simulink model "pv_panel_buck_converter_graphic"  (R2021a)
settings: Solver=VariableStepAuto  StartTime=0.0  StopTime=22  RelTol=1e-3  AbsTol=1e-3
libraries: spsSeriesRLCBranchLib x4, spsCurrentMeasurementLib x3, simulink x3, spsDiodeLib x1, spsMosfetLib x1, spsPVArrayLib x1, spsVoltageMeasurementLib x1, spspowerguiLib x1
settings Model: Creator=Uranus  LastModifiedBy=Uranus
settings SolverCC: AutoScaleAbsTol=off  AlgebraicLoopSolver=TrustRegion
settings DebuggingCC: SymbolicDimsDataTypeCodeGenerationDiagnostic=none  SFMachineParentedDataDiag=warning
settings SFSimCC: CustomCodeUndefinedFunction=UseInterfaceOnly
settings SimscapeCC: SimscapeLogType=all  SimscapeLogSimulationStatistics=on  SimscapeLogDataHistory=10000

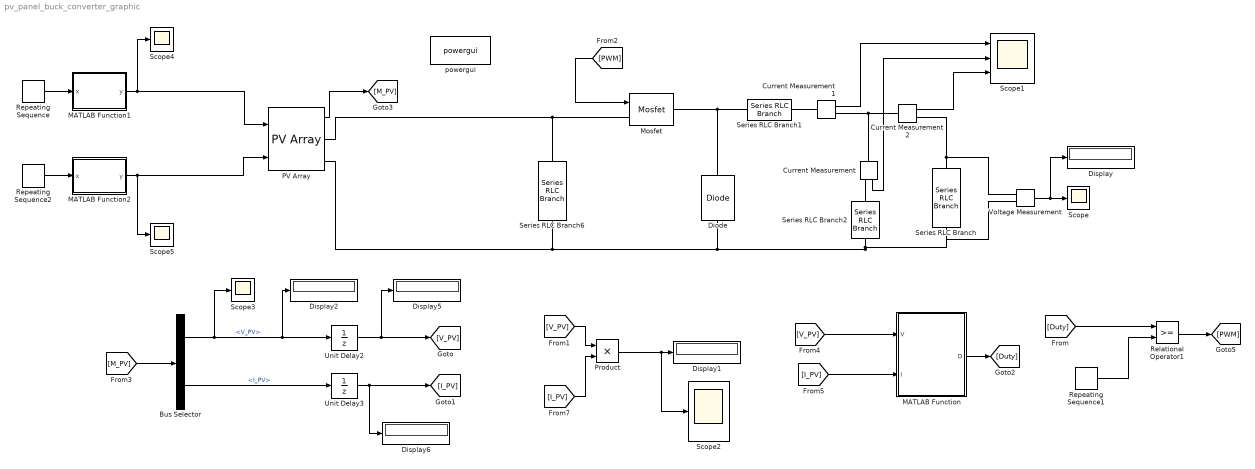
== system pv_panel_buck_converter_graphic ==
  Bus Selector : BusSelector  OutputSignals=V_PV,I_PV
  Current Measurement : spsCurrentMeasurementLib/Current Measurement  PhasorSimulation=off  OutputType=Complex  PSBequivalent=0
  Current Measurement1 : spsCurrentMeasurementLib/Current Measurement  PhasorSimulation=off  OutputType=Complex  PSBequivalent=0
  Current Measurement2 : spsCurrentMeasurementLib/Current Measurement  PhasorSimulation=off  OutputType=Complex  PSBequivalent=0
  Diode : spsDiodeLib/Diode  Ron=0.001  Lon=0  Vf=0.8  IC=0  UseSnubber=0  Rs=500  Cs=250e-9  Measurements=off
  Display{,1..2,5..6} (5 alike) : Display
  MATLAB Function : MATLAB Function  TreatAsAtomicUnit=on
  MATLAB Function1 : MATLAB Function  TreatAsAtomicUnit=on
  MATLAB Function2 : MATLAB Function  TreatAsAtomicUnit=on
  Mosfet : spsMosfetLib/Mosfet  Ron=0.0001  Lon=0  Rd=0.001  Vfd=0  IC=0  Rs=1e5  Cs=inf  Measurements=off
  PV Array : spsPVArrayLib/PV Array  Npar=1  Nser=1  PlotType=array @ 1000 W/m2 & specified temperatures  S_vec="[ 1000  500  100 ]"  Temp_C_vec="[ 15 30  ]"  ModuleName=User-defined  PlotWhenSelected=off  Pm=9  Ncell=60  Voc=20  Isc=1.5  Vm=18  Im=0.5  beta_Voc_pc=-0.3616  alpha_Isc_pc=0.041492  beta_Voc=-0.07232  alpha_Isc=0.00062238  IL=1.5  I0=3.9949e-08  nI=1.0405  Rsh=36.0004  Rs=3.9996  RobustModel=off  RobustCellTemperature=313.3991  BAL=on  Tc=1e-6  Tfilter=5e-5
  Product : Product
  Relational Operator1 : RelationalOperator  OutDataTypeStr=boolean  RndMeth=Simplest
  Repeating Sequence : simulink/Sources/Repeating Sequence  rep_seq_t=[0 2 8 10]  rep_seq_y=[0 2 8 10]
  Repeating Sequence1 : simulink/Sources/Repeating Sequence  rep_seq_t=[0 0.00001]  rep_seq_y=[0 1]
  Repeating Sequence2 : simulink/Sources/Repeating Sequence  rep_seq_t=[0 2 8 10]  rep_seq_y=[0 2 8 10]
  Scope{,2..5} (5 alike) : Scope
  Scope1 : Scope  NumInputPorts=3
  Series RLC Branch : spsSeriesRLCBranchLib/Series RLC Branch  LConnTagsString=__new0  RConnTagsString=__new0  BranchType=R  Resistance=20  Inductance=1e-3  SetiL0=off  InitialCurrent=0  Capacitance=1e-6  Setx0=off  InitialVoltage=0  Measurements=None
  Series RLC Branch1 : spsSeriesRLCBranchLib/Series RLC Branch  LConnTagsString=__new0  RConnTagsString=__new0  BranchType=L  Resistance=1  Inductance=40e-6  SetiL0=off  InitialCurrent=0  Capacitance=1e-6  Setx0=off  InitialVoltage=0  Measurements=None
  Series RLC Branch2 : spsSeriesRLCBranchLib/Series RLC Branch  LConnTagsString=__new0  RConnTagsString=__new0  BranchType=C  Resistance=1  Inductance=1e-3  SetiL0=off  InitialCurrent=0  Capacitance=10.625e-6  Setx0=off  InitialVoltage=0  Measurements=None
  Series RLC Branch6 : spsSeriesRLCBranchLib/Series RLC Branch  LConnTagsString=__new0  RConnTagsString=__new0  BranchType=RC  Resistance=1  Inductance=1e-3  SetiL0=off  InitialCurrent=0  Capacitance=1.5e-6  Setx0=off  InitialVoltage=0  Measurements=None
  Unit Delay2 : UnitDelay  SampleTime=1e-4  HasFrameUpgradeWarning=on
  Unit Delay3 : UnitDelay  SampleTime=1e-4  HasFrameUpgradeWarning=on
  Voltage Measurement : spsVoltageMeasurementLib/Voltage Measurement  PhasorSimulation=off  OutputType=Complex  PSBequivalent=0
  powergui : spspowerguiLib/powergui  Priority=1  SimulationMode=Continuous  SampleTime=50e-6  frequency=60  Iterations=50  frequencyindice=0  Pbase=100e6  ErrMax=1e-4  UnitsV=kV  UnitsW=MW  buscounter=0  FunctionMessages=off  echomessages=off  EnableUseOfTLC=off  CurrentSourceSwitches=off  DisableSnubberDevices=off  DisableRonSwitches=off  DisableVfSwitches=off  DisplayEquations=off  AutomaticDiscreteSolvers=off  SolverType=Tustin/Backward Euler (TBE)  Interpol=off  ExternalGateDelay=off  methode=off  Ts=100  x0status=blocks  SPID=on  SwTol=0  HookPort=off  NonlinearTolerance=1e-4  nMaxIteration=100  ContinueOnMaxIteration=off  RestoreLinks=warning  ResistiveCurrentMeasurement=off  Frange=[0:2:500]  Ylog=off  Xlog=on  ShowGrid=off  save=off  variable=ZData  structure=0  ZoomFFT=off  StartTime=0.0  cycles=1  DisplayStyle=1  fundamental=60  FreqAxis=off  MaxFrequency=1000  frequencyindicesteady=1  RmsSteady=1  display=off
  wires:
  Current Measurement1/1 -> Scope1/1
  Current Measurement/1 -> Scope1/2
  Current Measurement2/1 -> Scope1/3
  Voltage Measurement/1 -> Display/1, Scope/1
  PV Array/1 -> [M_PV]
  [PWM] -> Mosfet/1
  Product/1 -> Scope2/1, Display1/1
  Unit Delay3/1 -> [I_PV], Display6/1
  [V_PV] -> Product/1
  [I_PV] -> Product/2
  Bus Selector/1 -> Display2/1, Unit Delay2/1, Scope3/1  "<V_PV>"
  Bus Selector/2 -> Unit Delay3/1  "<I_PV>"
  [M_PV] -> Bus Selector/1
  Unit Delay2/1 -> [V_PV], Display5/1
  [I_PV] -> MATLAB Function/2(I)
  MATLAB Function/1(D) -> [Duty]
  Relational Operator1/1 -> [PWM]
  Repeating Sequence1/1 -> Relational Operator1/2
  [V_PV] -> MATLAB Function/1(V)
  [Duty] -> Relational Operator1/1
  MATLAB Function1/1(y) -> PV Array/1, Scope4/1
  Repeating Sequence/1 -> MATLAB Function1/1(x)
  Repeating Sequence2/1 -> MATLAB Function2/1(x)
  MATLAB Function2/1(y) -> PV Array/2, Scope5/1
  connections:
  Mosfet/LConn1 -- Series RLC Branch6/LConn1 -- PV Array/RConn1
  Mosfet/RConn1 -- Diode/RConn1 -- Series RLC Branch1/LConn1
  Series RLC Branch2/RConn1 -- Voltage Measurement/LConn2 -- Series RLC Branch/RConn1 -- Diode/LConn1 -- Series RLC Branch6/RConn1 -- PV Array/RConn2
  Current Measurement2/LConn1 -- Current Measurement/LConn1 -- Current Measurement1/RConn1
  Series RLC Branch2/LConn1 -- Current Measurement/RConn1
  Series RLC Branch/LConn1 -- Current Measurement2/RConn1 -- Voltage Measurement/LConn1
  Series RLC Branch1/RConn1 -- Current Measurement1/LConn1

== matlab function pv_panel_buck_converter_graphic/MATLAB Function ==
  data: V input; D output; I input
function D = MPPT_Algorithm (V,I) %D=MPPT output, V ile I=MPPT input
D_init = 0.66; %Duty cycle için ilk değer
D_max = 0.9;     %Duty cycle maximum değer
D_min = 0;       %Duty cycle minimum değer
deltaD = 1; %Duty cycle arttırmak/azaltmak için kullanılan artış değeri
persistent V_old P_old D_old;

if isempty(D_old)
    V_old=0;
    P_old=0;
    D_old=D_init;
end

%Güç hesaplaması:
P = V*I;
dV =V-V_old;
dP =P-P_old;

%P&O Algoritma yapısının kod yapısı:
if dP~=0
    if dP>0
        if dV>0
            D =D_old - deltaD;
        else 
            D =D_old + deltaD;
        end
    else
        if dV>0
            D =D_old + deltaD;
        else 
            D =D_old - deltaD;
        end
    end
else
    D = D_old;
end  
if D >= D_max || D<= D_min
    D = D_old;
end

%Güncellemeler yapılır:
D_old = D;
V_old = V;
P_old =P;

== matlab function pv_panel_buck_converter_graphic/MATLAB Function2 ==
  data: x input; y output
function y = fcn(x)

if x==0 
    y=15;
elseif x>0 && x<=2
    y=(15*x)/2+15;
elseif x>2 && x<=8
    y=30;
elseif x>8 && x<10
    y=(-15*x)/2+90;
else
    y=15;
end

== matlab function pv_panel_buck_converter_graphic/MATLAB Function1 ==
  data: x input; y output
function y = fcn(x)

if x>0 && x<2
    y=x*500;    
elseif x>=2 && x<=8
    y=1000;
elseif x>8 && x<10
    y=5000-500*x;

else 
    y=0;
end
